simulink model "simulationSprint2"  (R2018b)
settings: Solver=FixedStepAuto  StartTime=0.0  StopTime=10  FixedStep=0.01  MaxStep=100e-3  RelTol=1e-3
(part 2 of 3)

== stateflow chart simulationSprint2/Req6 and Req 7 ==
  note: The module responsible by test the requeriment six and seven.
      |
      | Notice : i_ means input signals
      | 		o_ means output signals
      |
      | Input :
      | i_enable - Start the test. 1- Start test . 0 - Do nothing.
      | i_desiredTest - Test Number Value. All the modules recieve the
      | signal and decide either execute the test. Ex: Value "1" means that will being testing the requeriment 1.
      | i_HeadLamp - State the Head Lamp. 1 - Light On ; 0 - Light Off.
      |
      |
      | Output :
      | o_TestResult - Result of test. 1 - Test ran correctly ; 2 - Test ran incorrectly.
      | o_TestDone - Test has been completed. 1 - Completed ;
      | o_keyfob - Signal that indicates if the key is inside or not from the car. 1 - Key inside ; 0 - Key outside.
      | o_keyCommand - Signal to lock or unlock the car. "1 - lock the car ; 0 - Unlock the car" ;  -1 - Do nothing.
      | o_startButtom - Signal to start or off the car. 1- Car Start ; 0 - Car off.
      | o_gear = gear State ; 1 - Park ; 0 - Engaged.
      | o_Door = Signal to generate the open or close door. 1 - Open Door ; 0 - Close Door.
  state state_OverHeadTest1
    during:
    o_keyCommand = 0;
    o_keyfob =1 ;
    o_gear = 1 ;
    o_door = 0;
    on after(100,msec):
    o_startButtom = 1;
    on after(2.5,sec):
    r_aux=1;
    exit :
    r_aux=0;
  state state_OverHeadTest
    during:
    o_keyCommand = 0;
    o_keyfob =1 ;
    o_startButtom = 0;
    on after(600,msec):
    r_aux=1;
    exit :
    r_aux=0;
  state state_OverHeadTest2
    during:
    o_startButtom = 0;
    on after(100,msec):
    o_keyCommand = 0;
    o_keyfob =1;
    on after(200,msec):
    r_aux=1;
    exit :
    r_aux=0;
    o_keyfob =0;
  state state_OverHeadTestReq7 [commented out]
    entry :
    r_aux2 = 0;
    r_aux=0;
    during:
    on after(2,sec):
    o_gear = 1 ;
    on after(2.2,sec):
    o_keyfob =1;
    on after(2.3,sec):
    o_keyCommand = 0;
    o_startButtom = 1;
    on after(2.8,sec):
    o_startButtom = 0;
    o_keyfob =0;
    on after(5.5,sec):
    r_aux2 = 1;
    on after(10,sec):
    r_aux=1;
    exit :
    r_aux=0;
    r_aux2=0;
  state state_idle
    during:
    r_aux =0;
    o_startButtom = 0;
    o_keyCommand = 1;
    o_keyfob =0;
  state State_error
    during:
    o_TestResult =0;
    o_testDone =1 ;
    on after(100,msec):
    r_aux =1;
    exit :
    r_aux =0;
  state State_feat_ok
    during:
    o_TestResult =1;
    o_testDone =1;
    on after(10,msec):
    r_aux =1;
    exit:
    r_aux =0;
  state status_req7
    during :
    on after(1,sec):
    if(i_HeadLamp ==0 )
    r_aux = 1;
    end
    exit :
    r_aux = 0;
  state state_update
    entry:
    r_aux = 0;
    during:
    o_TestResult =0;
    o_testDone = 0;
    r_aux =1 ;
    exit:
  (default) -> state_idle
  state_OverHeadTest -> state_OverHeadTest1 [order 2] : [r_aux==1 && i_HeadLamp==1 ]
  state_OverHeadTest1 -> state_OverHeadTest2 [order 2] : [r_aux==1 && i_HeadLamp==0]
  state_idle -> state_OverHeadTest : [i_enable ==1 && (i_DesiredTest==6 || i_DesiredTest==7)]
  state_update -> state_idle : [r_aux ==1]
  state_OverHeadTest1 -> State_error [order 1] : [r_aux==1 && i_HeadLamp==1]
  state_OverHeadTest -> State_error [order 1] : [r_aux==1 && i_HeadLamp==0 ]
  state_OverHeadTest2 -> status_req7 : [r_aux==1 && i_HeadLamp==0]
  status_req7 -> State_error [order 1] : [~after(10,sec) && r_aux==1]
  State_error -> state_update : [r_aux==1]
  State_feat_ok -> state_update : [r_aux==1]
  status_req7 -> State_feat_ok [order 2] : [after(10.5,sec) && i_HeadLamp ==0  ]
  data: i_enable input; i_DesiredTest input; o_TestResult output; o_testDone output; r_aux local; i_HeadLamp input; o_keyCommand output; o_keyfob output; o_startButtom output; r_aux2 local; o_gear output; o_door output

== stateflow chart simulationSprint2/Req9 ==
  note: The module responsible by test the requeriment nine.
      |
      | Notice : i_ means input signals
      | 		o_ means output signals
      |
      | Input :
      | i_enable - Start the test. 1- Start test . 0 - Do nothing.
      | i_desiredTest - Test Number Value. All the modules recieve the
      | signal and decide either execute the test. Ex: Value "1" means that will being testing the requeriment 1.
      | i_MotorState. 1 - On ; 0 - Off .
      |
      |
      | Output :
      | o_TestResult - Result of test. 1 - Test ran correctly ; 2 - Test ran incorrectly.
      | o_TestDone - Test has been completed. 1 - Completed ;
      | o_keyfob - Signal that indicates if the key is inside or not from the car. 1 - Key inside ; 0 - Key outside.
      | o_keyCommand - Signal to lock or unlock the car. "1 - lock the car ; 0 - Unlock the car" ;  -1 - Do nothing.
      | o_startButtom - Signal to start or off the car. 1- Car Start ; 0 - Car off.
      | o_gear = gear State ; 1 - Park ; 0 - Engaged.
  state state_testTurnOnCar
    during:
    o_keyfobcommand = 0;
    o_keyfob =1;
    o_gear = 1;
    on after(1,sec):
    o_startButtom = 1;
    on after(2,sec):
    r_aux=1;
    exit:
    r_aux = 0 ;
    o_startButtom = 0;
  state state_idle
    entry :
    r_aux = 0 ;
    o_keyfobcommand = 0;
    o_keyfob =0;
    o_gear = 0;
    on after(100,msec):
    o_startButtom = 0;
  state state_testTurnOffCar
    during:
    on after (100,msec):
    o_keyfob =0;
    o_keyfobcommand = 0;
    o_keyfob =0;
    o_gear = 1;
    on after(1.1,sec):
    o_startButtom = 1;
    on after(2,sec):
    r_aux=1;
    exit:
    r_aux = 0 ;
    o_startButtom = 0;
    o_keyfob =0;
  state State_error
    entry :
    during:
    o_TestResult =0;
    o_testDone =1 ;
    on after(200,msec):
    r_aux =1;
    exit :
    r_aux =0;
  state State_feat_ok
    entry :
    during:
    o_TestResult =1;
    o_testDone =1;
    o_startButtom=0;
    on after(200,msec):
    r_aux =1;
    exit:
    r_aux =0;
  state state_update
    entry:
    r_aux = 0;
    during:
    on after(1,sec):
    o_TestResult =0;
    o_testDone = 0;
    r_aux =1 ;
    exit:
  (default) -> state_idle
  state_idle -> state_testTurnOnCar : [i_enable==1 && i_desiredTest == 9 ]
  state_update -> state_idle : [r_aux ==1]
  state_testTurnOnCar -> State_error [order 2] : [r_aux==1 && i_motorState==0]
  state_testTurnOnCar -> state_testTurnOffCar [order 1] : [r_aux==1 && i_motorState==1]
  state_testTurnOffCar -> State_error [order 2] : [r_aux==1 && i_motorState==1]
  state_testTurnOffCar -> State_feat_ok [order 1] : [r_aux==1 && i_motorState==0]
  State_error -> state_update : [r_aux==1]
  State_feat_ok -> state_update : [r_aux==1]
  data: i_enable input size=1; i_desiredTest input int8 size=1; o_TestResult output int8 size=1; o_testDone output int8 size=1; r_aux local; i_motorState input int8 size=1; o_gear output int8 size=1; o_keyfob output int8 size=1; o_keyfobcommand output int8 size=1; o_startButtom output int8 size=1

== stateflow chart simulationSprint2/Req10 ==
  note: The module responsible by test the requeriment ten.
      |
      | Notice : i_ means input signals
      | 		o_ means output signals
      |
      | Input :
      | i_enable - Start the test. 1- Start test . 0 - Do nothing.
      | i_desiredTest - Test Number Value. All the modules recieve the
      | signal and decide either execute the test. Ex: Value "1" means that will being testing the requeriment 1.
      | i_RearLamps. 1 - Light On ; 0 - Light Off .
      |
      |
      | Output :
      | o_TestResult - Result of test. 1 - Test ran correctly ; 2 - Test ran incorrectly.
      | o_TestDone - Test has been completed. 1 - Completed ;
      | o_keyfob - Signal that indicates if the key is inside or not from the car. 1 - Key inside ; 0 - Key outside.
      | o_keyCommand - Signal to lock or unlock the car. "1 - lock the car ; 0 - Unlock the car" ;  -1 - Do nothing.
      | o_brake. 1- Breaking. 0 - Not Breaking.
  state state_RearLampCarOff
    entry :
    r_aux=0;
    during :
    o_keyfobcom = 0 ;
    o_keyfob = 0 ;
    on after(200,msec):
    o_brake =1 ;
    on after(600,msec):
    r_aux=1;
    exit:
    r_aux =0 ;
  state state_RearLampCarOn
    entry :
    r_aux=0;
    o_brake=0;
    during :
    o_keyfobcom = 0 ;
    o_keyfob = 1 ;
    on after(200,msec):
    o_brake =1 ;
    on after(700,msec):
    r_aux=1;
    exit:
    r_aux =0 ;
    o_brake =0 ;
    o_keyfob = 0 ;
  state state_idle
    entry :
    r_aux=0;
  state State_error
    during:
    o_TestResult =0;
    o_testDone =1 ;
    on after(100,msec):
    r_aux =1;
    exit :
    r_aux =0;
  state State_feat_ok
    during:
    o_TestResult =1;
    o_testDone =1;
    on after(100,msec):
    r_aux =1;
    exit:
    r_aux =0;
  state state_update
    entry:
    r_aux = 0;
    on after(500,msec):
    during:
    o_TestResult =0;
    o_testDone = 0;
    r_aux =1 ;
    exit:
  (default) -> state_idle
  state_idle -> state_RearLampCarOff : [i_enable==1 && i_desiredTest==10]
  state_RearLampCarOff -> state_RearLampCarOn [order 1] : [r_aux==1 && i_RearLamps==0]
  state_RearLampCarOff -> State_error [order 2] : [r_aux==1 && i_RearLamps==1]
  state_update -> state_idle : [r_aux==1]
  state_RearLampCarOn -> State_error [order 2] : [r_aux==1 && i_RearLamps==0]
  state_RearLampCarOn -> State_feat_ok [order 1] : [r_aux==1 && i_RearLamps==1]
  State_error -> state_update : [r_aux==1]
  State_feat_ok -> state_update : [r_aux==1]
  data: i_enable input; i_desiredTest input; i_RearLamps input; o_TestResult output; o_testDone output; r_aux local; o_brake output; o_keyfob output; o_keyfobcom output

== stateflow chart simulationSprint2/Req12 ==
  note: The module responsible by test the requeriment twelve.
      |
      | Notice : i_ means input signals
      | 		o_ means output signals
      |
      | Input :
      | i_enable - Start the test. 1- Start test . 0 - Do nothing.
      | i_desiredTest - Test Number Value. All the modules recieve the
      | signal and decide either execute the test. Ex: Value "1" means that will being testing the requeriment 1.
      | i_IPCInd. 0 - Showing nothing ; 1 - Showing items .
      | i_batteryLevel . Containg the battery level value. Range = 0 - 100 %
      | i_batterySocWarning. Warning of low Battery level . If the battery value for less than or equal to 10%
      |
      | Output :
      | o_TestResult - Result of test. 1 - Test ran correctly ; 2 - Test ran incorrectly.
      | o_TestDone - Test has been completed. 1 - Completed ;
      | o_keyfob - Signal that indicates if the key is inside or not from the car. 1 - Key inside ; 0 - Key outside.
      | o_keyCommand - Signal to lock or unlock the car. "1 - lock the car ; 0 - Unlock the car" ;  -1 - Do nothing.
      | o_doorCom - Signal to represent the opening the door. 1 - Opening ; 0 - Closing ; -1 - Do nothing.
  state state_ipcoff
    during :
    o_keyfobcom = 0;
    o_keyfob = 0;
    on after(200,msec):
    r_aux=1;
    exit:
    r_aux =0;
  state state_idle
    entry:
    r_aux=0;
  state state_ipcOn
    during :
    o_keyfobcom = 0;
    o_keyfob = 1;
    on after(500,msec):
    o_doorCom = 1;
    on after(1,sec):
    r_aux=1;
    exit:
    r_aux =0;
    o_doorCom = 0;
  state State_error
    during:
    o_TestResult =0;
    o_testDone =1 ;
    on after(300,msec):
    r_aux =1;
    exit :
    r_aux =0;
    o_keyfob = 0;
  state state_batteryLevel
    during :
  state State_feat_ok
    entry :
    o_keyfob = 0;
    during:
    o_TestResult =1;
    o_testDone =1;
    on after(500,msec):
    r_aux =1;
    exit:
    r_aux =0;
    o_keyfob = 0;
  state state_update
    entry:
    r_aux = 0;
    during:
    on after(200,msec):
    o_TestResult =0;
    o_testDone = 0;
    r_aux =1 ;
    exit:
  (default) -> state_idle
  state_idle -> state_ipcoff : [i_enable==1 && i_desiredTest == 12 ]
  state_ipcoff -> State_error [order 2] : [r_aux==1 && i_IPCInd==1]
  state_update -> state_idle : [r_aux==1]
  state_ipcoff -> state_ipcOn [order 1] : [r_aux==1 && i_IPCInd==0]
  state_ipcOn -> State_error [order 2] : [r_aux==1 && i_IPCInd==0]
  State_error -> state_update : [r_aux==1]
  state_batteryLevel -> State_error [order 2] : [((i_batteryLevel <=10 && i_batterySocWarning==0 ) || (i_batteryLevel >10 && i_batterySocWarning==1 )) && after(500,msec)  ]
  state_ipcOn -> state_batteryLevel [order 1] : [r_aux==1 && i_IPCInd==1]
  state_batteryLevel -> State_feat_ok [order 1] : [((i_batteryLevel <=10 && i_batterySocWarning==1 ) || (i_batteryLevel >10 && i_batterySocWarning==0 )) && after(500,msec)  ]
  State_feat_ok -> state_update : [r_aux==1]
  data: i_enable input; i_desiredTest input; o_TestResult output; o_testDone output; r_aux local; i_IPCInd input; o_keyfob output; o_keyfobcom output; o_doorCom output; i_batteryLevel output; i_batterySocWarning input

== stateflow chart simulationSprint2/Req13 ==
  note: The module responsible by test the requeriment thirteen.
      |
      | Notice : i_ means input signals
      | 		o_ means output signals
      |
      | Input :
      | i_enable - Start the test. 1- Start test . 0 - Do nothing.
      | i_desiredTest - Test Number Value. All the modules recieve the
      | signal and decide either execute the test. Ex: Value "1" means that will being testing the requeriment 1.
      | i_ajarDoor. 1 - Door in aja state  ; 0 -  Door not in aja state .
      |
      |
      | Output :
      | o_TestResult - Result of test. 1 - Test ran correctly ; 0 - Test ran incorrectly.
      | o_TestDone - Test has been completed. 1 - Completed ;
      | o_keyCommand - Signal to lock or unlock the car. "1 - lock the car ; 0 - Unlock the car" ;  -1 - Do nothing.
      | o_doorajar. Signal to represent the opening the door. 1 - Opening ; 0 - Closing ; -1 - Do nothing.
  state state_testajarDoorTrue
    during:
    o_keyfobcommand = 0;
    o_doorAjar = 1;
    on after(200,msec):
    r_aux=1;
    exit:
    r_aux=0;
  state state_testajarDoorTrue1
    during:
    o_keyfobcommand = 0;
    o_doorAjar = 0;
    on after(500,msec):
    r_aux=1
    exit:
    r_aux=0;
  state state_idle
    entry:
    r_aux=0;
    o_doorAjar = 0;
    o_keyfobcommand = 0;
  state state_testCarlock
    during:
    o_keyfobcommand = 1;
    o_doorAjar = 1;
    on after(1,sec):
    r_aux=1
    exit:
    r_aux=0;
  state State_error
    during:
    o_TestResult =0;
    o_testDone =1 ;
    on after(100,msec):
    r_aux =1;
    exit :
    r_aux =0;
    o_doorAjar = 0;
  state State_feat_ok
    during:
    o_TestResult =1;
    o_testDone =1;
    on after(100,msec):
    r_aux =1;
    exit:
    r_aux =0;
  state state_update
    entry:
    r_aux = 0;
    on after(5,msec):
    during:
    o_TestResult =0;
    o_testDone = 0;
    r_aux =1 ;
    exit:
  state_testajarDoorTrue -> state_testajarDoorTrue1 [order 2] : [r_aux==1 && i_doorAjar == 1]
  state_testajarDoorTrue -> State_error [order 1] : [r_aux==1 && i_doorAjar == 0]
  (default) -> state_idle
  state_idle -> state_testajarDoorTrue : [i_enable==1 && i_desiredTest == 13 ]
  state_testajarDoorTrue1 -> State_error [order 2] : [r_aux==1 && i_doorAjar == 1]
  state_update -> state_idle : [r_aux==1]
  state_testajarDoorTrue1 -> state_testCarlock [order 1] : [r_aux==1 && i_doorAjar == 0]
  state_testCarlock -> State_error [order 2] : [r_aux==1 && i_doorAjar == 1]
  State_error -> state_update : [r_aux==1]
  state_testCarlock -> State_feat_ok [order 1] : [r_aux==1 && i_doorAjar == 0]
  State_feat_ok -> state_update : [r_aux==1]
  data: i_enable input; i_desiredTest input; i_doorAjar input; o_TestResult output; o_testDone output; r_aux local; o_doorAjar output int8; o_keyfobcommand output

== stateflow chart simulationSprint2/Req15 ==
  note: The module responsible by test the requeriment fifteen.
      |
      | Notice : i_ means input signals
      | 		o_ means output signals
      |
      | Input :
      | i_enable - Start the test. 1- Start test . 0 - Do nothing.
      | i_desiredTest - Test Number Value. All the modules recieve the
      | signal and decide either execute the test. Ex: Value "1" means that will being testing the requeriment 1.
      | i_gear -  geared State ; 1 - Park ; 0 - Engaged.
      | i_MotorStatus. 1 - On ; 0 - Off .
      |
      |
      | Output :
      |
      | o_TestResult - Result of test. 1 - Test ran correctly ; 0 - Test ran incorrectly.
      | o_TestDone - Test has been completed. 1 - Completed ;
      | o_keyComm - Signal to lock or unlock the car. "1 - lock the car ; 0 - Unlock the car" ;  -1 - Do nothing.
      | o_startButtom - Signal to start or off the car. 1- Car Start ; 0 - Car off.
      | o_keyfob - Signal that indicates if the key is inside or not from the car. 1 - Key inside ; 0 - Key outside.
      | o_gear = gear State ; 1 - Park ; 0 - Engaged.
  state state_gearParkOffCar
    entry:r_aux=0;
    during:
    o_keyfobcom = 0;
    on after(200,msec):
    o_keyfob =1;
    o_gear=1;
    on after(1,sec):
    o_startButtom =1;
    on after(2,sec):
    r_aux=1;
    exit :
    r_aux=0;
  state state_idle
    entry:
    r_aux=0;
  state State_error
    during:
    o_TestResult =0;
    o_testDone =1 ;
    on after(200,msec):
    r_aux =1;
    exit :
    r_aux =0;
  state state_gearParkOnCar
    entry:r_aux=0;
    during:
    o_keyfobcom = 0;
    on  after(200,msec):
    o_keyfob =1;
    o_gear=0;
    on after(400,msec):
    o_startButtom =0;
    on after(1,sec):
    r_aux=1;
    exit :
    r_aux=0;
  state state_update
    entry:
    r_aux = 0;
    on after(400,msec):
    during:
    o_TestResult =0;
    o_testDone = 0;
    r_aux =1 ;
    exit:
    o_keyfobcom = 0;
    o_keyfob =0;
    o_gear=0;
  state State_feat_ok
    during:
    o_TestResult =1;
    o_testDone =1;
    on after(200,msec):
    r_aux =1;
    exit:
    r_aux =0;
  state state_gear
    during :
    o_gear = 1;
    o_startButtom =0;
  (default) -> state_idle
  state_idle -> state_gearParkOffCar : [i_enable==1 && i_desiredTest == 15]
  state_gearParkOffCar -> state_gearParkOnCar [order 1] : [r_aux==1 && i_motorStatus==1 && i_gear ==1]
  state_gearParkOffCar -> State_error [order 2] : [(r_aux==1 && i_motorStatus==0) || (r_aux==1 && i_gear ~=1) ]
  state_update -> state_idle : [r_aux==1]
  state_gear -> State_error [order 2] : [after(500,msec) &&  i_motorStatus==1]
  state_gearParkOnCar -> State_error [order 2] : [r_aux==1 && i_motorStatus==0]
  State_error -> state_update : [r_aux==1]
  state_gearParkOnCar -> state_gear [order 1] : [r_aux==1 && i_motorStatus==1]
  state_gear -> State_feat_ok [order 1] : [after(500,msec)  && i_motorStatus==0]
  State_feat_ok -> state_update : [r_aux==1]
  data: i_enable input; i_desiredTest input; o_TestResult output; o_testDone output; r_aux local; i_motorStatus input; o_gear output; o_keyfob output; o_keyfobcom output; o_startButtom output; i_gear input

== stateflow chart simulationSprint2/Req16 ==
  note: The module responsible by test the requeriment sixteen.
      |
      | Notice : i_ means input signals
      | 		o_ means output signals
      |
      | Input :
      | i_enable - Start the test. 1- Start test . 0 - Do nothing.
      | i_desiredTest - Test Number Value. All the modules recieve the
      | signal and decide either execute the test. Ex: Value "1" means that will being testing the requeriment 1.
      | i_MotorStatus. 1 - On ; 0 - Off .
      | i_headLampLowBeam. 1 - Lamp  On ; 0 - Lamp Off.
      | i_headLampPark. 1 - Lamp On ; 0 - Lamp Off.
      | i_headLampHigh. 1 - Lamp On ; 0 - Lamp Off.
      |
      |
      | Output :
      | o_TestResult - Result of test. 1 - Test ran correctly ; 2 - Test ran incorrectly.
      | o_TestDone - Test has been completed. 1 - Completed ;
      | o_keyfobComm - Signal to lock or unlock the car. "1 - lock the car ; 0 - Unlock the car" ;  -1 - Do nothing.
      | o_headLamp - Light mode.
      | o_startButtom - Signal to start or off the car. 1- Car Start ; 0 - Car Off.
      | o_keyfob - Signal that indicates if the key is inside or not from the car. 1 - Key inside ; 0 - Key outside.
      | o_levelluminosity - Luminosity Level. Range 0 ~ 4.
  state StateTurnOnCar
    during :
    o_keyfobCom = 0;
    on after(50,msec):
    o_keyfob = 1;
    on after(100,msec):
    o_gear = 1;
    o_headLamp = 0;
    on after(150,msec):
    o_startButtom = 1;
  state state_tryTurnDown_Car
    during :
    o_startButtom = 0;
  state state_tryTurnDown_Car2
    during :
    o_headLamp = 0;
  state stateTurnOnHeadLamp
    during :
    o_headLamp = 1;
  state state_idle1
    entry:
    r_aux=0;
    o_keyfob = 0 ;
    o_levelluminosity = 4;
  state State_error1
    during:
    o_TestResult =0;
    o_testDone =1 ;
    on after(200,msec):
    r_aux =1;
    exit :
    r_aux =0;
  state state_update1
    entry:
    r_aux = 0;
    on after(200,msec):
    during:
    o_TestResult =0;
    o_testDone = 0;
    r_aux =1 ;
    exit:
    o_keyfob = 0;
    o_keyfobCom = 0;
    o_headLamp=0;
    o_startButtom = 0;
  state State_feat_ok1
    during:
    o_TestResult =1;
    o_testDone =1;
    on after(200,msec):
    r_aux =1;
    exit:
    r_aux =0;
  (default) -> state_idle1
  state_tryTurnDown_Car -> state_tryTurnDown_Car2 [order 2] : [after(1,sec) && i_motorStatus ==1]
  StateTurnOnCar -> stateTurnOnHeadLamp [order 2] : [after(300,msec) && i_motorStatus==1]
  stateTurnOnHeadLamp -> state_tryTurnDown_Car [order 1] : [after(100,msec) && i_headLampPark == 1 && i_headLampLowBeam == 0 ]
  state_update1 -> state_idle1 : [r_aux==1]
  state_idle1 -> StateTurnOnCar : [i_enable==1 && i_desiredTest ==16]
  stateTurnOnHeadLamp -> State_error1 [order 2] : [after(100,msec) && i_headLampPark ~= 1 && i_headLampLowBeam ~= 0 ]
  state_tryTurnDown_Car2 -> State_error1 [order 2] : [after(500,msec) && i_motorStatus ==1]
  state_tryTurnDown_Car2 -> State_feat_ok1 [order 1] : [after(500,msec) && i_motorStatus ==0]
  state_tryTurnDown_Car -> State_error1 [order 1] : [after(1,sec) && i_motorStatus ==0]
  StateTurnOnCar -> State_error1 [order 1] : [after(300,msec) && i_motorStatus==0]
  State_error1 -> state_update1 : [r_aux==1]
  State_feat_ok1 -> state_update1 : [r_aux==1]
  data: i_enable input; i_desiredTest input; o_TestResult output; o_testDone output; r_aux local; o_keyfobCom output; o_startButtom output; o_keyfob output; o_headLamp output; i_motorStatus input; i_headLampPark input; i_headLampLowBeam input; i_headLampHigh input; o_levelluminosity output double; o_gear output

== stateflow chart simulationSprint2/Req17 ==
  note: The module responsible by test the requeriment seventeen.
      |
      | Notice : i_ means input signals
      | 		o_ means output signals
      |
      | Input :
      | i_enable - Start the test. 1- Start test . 0 - Do nothing.
      | i_desiredTest - Test Number Value. All the modules recieve the
      | signal and decide either execute the test. Ex: Value "1" means that will being testing the requeriment 1.
      | i_lampValue. 1- Turn Lamp On ; 0 - Turn Lamp Off .
      |
      |
      | Output :
      | o_TestResult - Result of test. 1 - Test ran correctly ; 2 - Test ran incorrectly.
      | o_TestDone - Test has been completed. 1 - Completed ;
      | o_keyfobComm - Signal to lock or unlock the car. "1 - lock the car ; 0 - Unlock the car" ;  -1 - Do nothing.
      | o_keyfob - Signal that indicates if the key is inside or not from the car. 1 - Key inside ; 0 - Key outside.
  state state_testBlinkUnlockTheCar
    entry: r_aux = 0;
    during :
    on after(5,sec):
    o_keyfobcom = 0;
    on after(5.1,sec):
    if (i_lamp_value ~=r_lamp_value )
    r_blink = r_blink +1;
    r_lamp_value = i_lamp_value ;
    end
    exit:
    r_blink  = 0;
  state state_idle
    entry:
    r_aux=0;
    r_lamp_value = i_lamp_value ;
    o_ketfob = 0;
    o_keyfobcom = 1;
    r_blink = 0;
  state state_testBlinkUnlockTheCar1
    entry: r_aux = 0;
    r_lamp_value = i_lamp_value;
    during :
    o_keyfobcom = 1;
    if (i_lamp_value ~=r_lamp_value )
    r_blink = r_blink +1;
    r_lamp_value = i_lamp_value ;
    end
  state State_feat_ok
    during:
    o_TestResult =1;
    o_testDone =1;
    on after(200,msec):
    r_aux =1;
    exit:
    r_aux =0;
  state State_error
    during:
    o_TestResult =0;
    o_testDone =1 ;
    on after(200,msec):
    r_aux =1;
    exit :
    r_aux =0;
  state state_update
    entry:
    r_aux = 0;
    on after(500,msec):
    during:
    o_TestResult =0;
    o_testDone = 0;
    r_aux =1 ;
    exit:
    o_keyfobcom = 0;
  (default) -> state_idle
  state_idle -> state_testBlinkUnlockTheCar : [i_enable==1 && i_desiredTest ==17  ]
  state_testBlinkUnlockTheCar -> state_testBlinkUnlockTheCar1 [order 1] : [after(30,sec) && r_blink==2]
  state_update -> state_idle : [r_aux==1]
  state_testBlinkUnlockTheCar -> State_error [order 2] : [after(26,sec) && r_blink~=2]
  state_testBlinkUnlockTheCar1 -> State_error [order 2] : [after(40,sec) && r_blink~=4]
  state_testBlinkUnlockTheCar1 -> State_feat_ok [order 1] : [after(40,sec) && r_blink==4]
  State_feat_ok -> state_update : [r_aux==1]
  State_error -> state_update : [r_aux==1]
  data: i_enable input int8; i_desiredTest input int8; o_TestResult output int8; o_testDone output int8; r_aux local; r_blink local; r_lamp_value local; i_lamp_value input int8; o_ketfob output int8; o_keyfobcom output int8

== stateflow chart simulationSprint2/Req18 ==
  note: The module responsible by test the requeriment nineteen.
      |
      | Notice : i_ means input signals
      | 		o_ means output signals
      |
      | Input :
      | i_enable - Start the test. 1- Start test . 0 - Do nothing.
      | i_desiredTest - Test Number Value. All the modules recieve the
      | signal and decide either execute the test. Ex: Value "1" means that will being testing the requeriment 1.
      | Car Lock State. 1- Unlock ; 0 - Lock .
      |
      |
      | Output :
      | o_TestResult - Result of test. 1 - Test ran correctly ; 2 - Test ran incorrectly.
      | o_TestDone - Test has been completed. 1 - Completed ;
      | o_keyfobComm - Signal to lock or unlock the car. "1 - lock the car ; 0 - Unlock the car" ;  -1 - Do nothing.
  state state_DrlOn
    entry :
    r_aux=0;
    during :
    on after(20,sec):
    o_keyfobcom = 0;
    on after(40,sec):
    r_aux = 1 ;
    exit :
    r_aux = 0;
  state state_DrlOff
    entry : r_aux=0;
    during :
    o_keyfobcom =1;
    on after(40,sec):
    r_aux = 1 ;
    exit :
    r_aux = 0 ;
  state state_idle
    entry:
    r_aux=0;
    o_keyfobcom = 1;
  state State_feat_ok
    during:
    o_TestResult =1;
    o_testDone =1;
    on after(200,msec):
    r_aux =1;
    exit:
    r_aux =0;
  state State_error
    during:
    o_TestResult =0;
    o_testDone =1 ;
    on after(200,msec):
    r_aux =1;
    exit :
    r_aux =0;
  state state_update
    entry:
    r_aux = 0;
    on after(300,msec):
    during:
    o_TestResult =-1;
    o_testDone = 0;
    r_aux =1 ;
    exit:
  (default) -> state_idle
  state_idle -> state_DrlOn : [i_enable==1 && i_desiredTest == 18 ]
  state_DrlOn -> state_DrlOff [order 1] : [r_aux==1 && i_DRL==1]
  state_DrlOn -> State_error [order 2] : [r_aux==1 && i_DRL==0]
  state_DrlOff -> State_error [order 2] : [r_aux==1 && i_DRL==1]
  state_DrlOff -> State_feat_ok [order 1] : [r_aux==1 && i_DRL==0]
  state_update -> state_idle : [r_aux==1]
  State_feat_ok -> state_update : [r_aux==1]
  State_error -> state_update : [r_aux==1]
  data: i_enable input int8; i_desiredTest input; o_TestResult output; o_testDone output; i_DRL input; r_aux local double; o_keyfobcom output

== stateflow chart simulationSprint2/"Req 2" ==
  note: The module responsible by test the requeriment one.
      |
      | Notice : i_ means input signals
      | 		o_ means output signals
      |
      | Input :
      | i_enable - Start the test. 1- Start test . 0 - Do nothing.
      | i_desiredTest - Test Number Value. All the modules recieve the
      | signal and decide either execute the test. Ex: Value "1" means that will being testing the requeriment 1.
      | i_WindowRightState = Windows State. 1- Windows Opening  ; 0 - Windows Closing ;  -1 - Do nothing.
      | i_WindowLeftState = Windows State. 1- Windows Opening  ; 0 - Windows Closing ;  -1 - Do nothing.
      | Output :
      | o_keyfob - Signal that indicates if the key is inside or not from the car. 1 - Key inside ; 0 - Key outside.
      | o_startButtom - Signal to start or off the car. 1- Car Start ; 0 - Car off.
      | o_WindowValue - Signal to move the windows " 1 - Opening ; 0- Closing ; -1 - Do Nothing  ;
      | o_gear = gear State ; 1 - Park ; 0 - Engaged.
      | o_keyfobCommand - Signal to lock or unlock the car. "1 - lock the car ; 0 - Unlock the car" ;  -1 - Do nothing.
      | o_TestResult - Result of test. 1 - Test ran correctly ; 2 - Test ran incorrectly.
      | o_TestDone - Test has been completed. 1 - Completed ;
  state State_idle
    exit :
    r_aux=0;
    r_count = 1 ;
    r_error = 0;
    o_startButtom = 0;
    o_keyfobCommand = 2;
    o_gear = 0 ;
    o_keyfob=0;
    o_WindowValue = -1;
  state state_readyingSystem
    during:
    on after (50,msec):
    o_keyfob =1;
    o_keyfobCommand = 0 ;
    o_gear = 1 ;
    on after(0.5,sec):
    o_startButtom = 1;
    on after(1.5,sec):
    r_aux=1;
    exit :
    r_aux=0;
  state state_testCarOn
    during:
    o_WindowValue =0 ;
    on after(2,sec):
    r_aux=1;
    exit :
    r_aux=0;
  state state_testCarOff
    during:
    o_startButtom = 0;
    on after(2,sec):
    o_WindowValue= 0;
    on after(3,sec):
    r_aux=1;
    exit :
    r_aux=0;
    o_WindowValue= -1;
  state State_error
    during:
    o_TestResult =0;
    o_testDone =1 ;
    on after(200,msec):
    r_aux =1;
    exit :
    r_aux =0;
  state state_temp
  state state_testAfter10sec
    entry:
    o_WindowValue= 0;
  state state_update
    entry:
    r_aux = 0;
    during:
    o_TestResult =0;
    o_testDone = 0;
    on after(500,msec):
    r_aux =1 ;
    exit:
  state State_feat_ok
    during:
    o_TestResult =1;
    o_testDone =1;
    on after(200,msec):
    r_aux =1;
    exit:
    r_aux =0;
  (default) -> State_idle
  State_idle -> state_readyingSystem : [i_enable==1 && i_desiredTest ==2 ]
  state_readyingSystem -> state_testCarOn : [r_aux==1]
  state_testCarOn -> state_testCarOff [order 2] : [(i_WindowRightState==0 && i_WindowLeftState == 0)  && r_aux==1]
  state_update -> State_idle : [r_aux==1]
  state_testCarOn -> State_error [order 1] : [(i_WindowRightState~=0 || i_WindowLeftState ~= 0)   && r_aux==1]
  state_testCarOff -> State_error [order 2] : [(i_WindowRightState~=0 || i_WindowLeftState ~= 0)   && r_aux==1]
  state_testAfter10sec -> State_error [order 1] : [(i_WindowRightState~=-1 && i_WindowLeftState ~= -1) && after(300,msec)]
  State_error -> state_update : [r_aux==1]
  state_testCarOff -> state_temp [order 1] : [(i_WindowRightState==0 && i_WindowLeftState == 0)  && r_aux==1]
  state_temp -> state_testAfter10sec : [after(11,sec)]
  state_testAfter10sec -> State_feat_ok [order 2] : [(i_WindowRightState==-1 && i_WindowLeftState == -1) && after(300,msec)]
  State_feat_ok -> state_update : [r_aux==1]
  data: o_TestResult output; r_aux local; i_desiredTest input; i_enable input; r_error local; o_testDone output; r_count local; o_keyfob output; i_WindowRightState input; o_keyfobCommand output; o_startButtom output; o_WindowValue output; o_gear output; i_WindowLeftState input

== stateflow chart simulationSprint2/Req 4 ==
  state state_test_unlock_doors [commented out]
    during:
    o_keyfob =1;
    o_keyfobCom = 0;
    on after(10,msec):
    o_lockDoor = 0 ;
    on after(1.5,sec):
    r_aux = 1;
    exit : r_aux = 0;
  note: The module responsible by test the requeriment four.
      |
      | Notice : i_ means input signals
      | 		o_ means output signals
      |
      | Input :
      | i_enable - Start the test. 1- Start test . 0 - Do nothing.
      | i_desiredTest - Test Number Value. All the modules recieve the
      | signal and decide either execute the test. Ex: Value "1" means that will being testing the requeriment 1.
      | i_WindowsStateAnd - And condition with the WindowState . 1-  Both is Windows Closing ; 0 - Windows Opening ;  -1 - Do nothing.
      | i_WindowsStateAnd - And condition with the DoorState. 1 - Both Door are closing  ;  0 - Some Door is opening ;  -1 Do nothing.
      | i_WindowsStateOr - Or condition with the DoorState. 1 - Some Door is closing ;  0 - Both Door are opening ;  -1 Do nothing.
      | i_stateDoorAnd - And condition with the Door Lock State. 1 - Both Door are Locked; 0 - Some Door is unlocked; -1 Do nothing.
      | i_stateDoorOR - Or condition with the Door Lock State. 1 - Some Door is locked;  0 - Both Door are unlocked ;  -1 Do nothing.
      |
      | Output :
      | o_TestResult - Result of test. 1 - Test ran correctly ; 2 - Test ran incorrectly.
      | o_TestDone - Test has been completed. 1 - Completed .
      | o_keyfob - Signal that indicates if the key is inside or not from the car. 1 - Key inside ; 0 - Key outside.
      | o_keyfobComm - Signal to lock or unlock the car. "1 - lock the car ; 0 - Unlock the car" ;  -1 - Do nothing.
      | o_WindowState - Signal to move the windows " 0 - Opening ; 1- Closing ; -1 - Do Nothing  ;
      | o_lockDoor = Lock Door ; 1 - Lock the doors; 0 - unlock the doors.
  state State_idle
    entry :
    r_aux=0;
    o_TestResult = 0;
    o_lockDoor=-1;
    during:
  state state_test_lock_doors
    during:
    o_keyfob =1;
    o_keyfobCom = 0;
    on after(200,msec):
    o_lockDoor = 1 ;
    on after(300,msec):
    o_gear =1;
    on after(400,msec):
    o_startButtom =1 ;
    on after(1.7,sec):
    r_aux = 1;
    exit : r_aux = 0;
  state state_test_windowsTest
    during:
    o_keyfob =1;
    o_keyfobCom = 0;
    on after(100,msec):
    o_startButtom =1 ;
    on after(600,msec):
    o_DDSCommand = 0;
    on after(1,sec):
    o_windowState = 0 ;
    on after(2.5,sec):
    r_aux = 1;
    exit : r_aux = 0;
  state State_error
    during:
    o_TestResult =0;
    o_testDone =1 ;
    on after(100,msec):
    r_aux =1;
    exit :
    r_aux =0;
  state state_WindowsTest1
    during:
    o_keyfob =1;
    o_keyfobCom = 0;
    on after(100,msec):
    o_startButtom =1 ;
    on after(800,msec):
    o_DDSCommand = 1;
    on after(2.4,sec):
    o_windowState = 1 ;
    on after(4,sec):
    r_aux = 1;
    exit : r_aux = 0;
  state State_feat_ok
    entry :
    o_lockDoor=0;
    o_keyfob = 0 ;
    o_keyfobCom =0;
    during:
    o_TestResult =1;
    o_testDone =1;
    on after(500,msec):
    r_aux =1;
    exit:
    r_aux =0;
  state state_update
    entry:
    o_lockDoor=0;
    o_keyfob = 0 ;
    o_keyfobCom =0;
    r_aux = 0;
    on after(500,msec):
    during:
    o_TestResult =0;
    o_testDone = 0;
  (default) -> ? [commented out] : [r_aux ==1 &&  i_stateDoorRight==0 && i_stateDoorLeft ==0]
  state_test_unlock_doors -> ? [commented out] : [r_aux ==1 &&  i_stateDoorRight ~=0 && i_stateDoorLeft ~=0]
  (default) -> State_idle
  State_idle -> state_test_lock_doors : [i_enable==1 && i_desiredTest ==4 ]
  state_test_lock_doors -> state_test_windowsTest [order 1] : [r_aux ==1 &&  i_stateDoorRight==1 && i_stateDoorLeft ==1]
  state_update -> State_idle : [after(100,msec)]
  state_test_windowsTest -> State_error [order 2] : [r_aux ==1 &&  i_windowStateLeft~=-1 && i_windowStateRight~=-1]
  state_test_lock_doors -> State_error [order 2] : [r_aux ==1 &&  i_stateDoorRight~=1 && i_stateDoorLeft ~=1]
  state_test_windowsTest -> state_WindowsTest1 [order 1] : [r_aux ==1 &&  i_windowStateLeft==-1 && i_windowStateRight==-1]
  state_WindowsTest1 -> State_error [order 2] : [r_aux ==1 &&  i_windowStateLeft~=1 && i_windowStateRight~=1]
  State_error -> state_update : [r_aux==1]
  state_WindowsTest1 -> State_feat_ok [order 1] : [r_aux ==1 &&  i_windowStateLeft==1 && i_windowStateRight==1]
  State_feat_ok -> state_update : [r_aux==1]
  data: o_TestResult output; r_aux local; i_desiredTest input; i_enable input; o_testDone output; i_stateDoorRight input; i_stateDoorLeft input; o_keyfob output; o_keyfobCom output; o_lockDoor output; o_windowState output; i_windowStateLeft input; o_startButtom output; o_DDSCommand output; i_windowStateRight input; o_gear output

== stateflow chart simulationSprint2/Req19 ==
  note: The module responsible by test the requeriment fourteen.
      |
      | Notice : i_ means input signals
      | 		o_ means output signals
      |
      | Input :
      | i_enable - Start the test. 1- Start test . 0 - Do nothing.
      | i_desiredTest - Test Number Value. All the modules recieve the
      | signal and decide either execute the test. Ex: Value "1" means that will being testing the requeriment 1.
      | i_MotorState. 1 - On ; 0 - Off .
      | i_speed - Car Speed. Range - 0 ~ 220 km/h
      | i_LeftBackDoorLockState. 1 - Door Unlock . 0 - Door Lock.
      | i_RightBackDoorLockState. 1 - Door Unlock . 0 - Door Lock.
      |
      | Output :
      | o_TestResult - Result of test. 1 - Test ran correctly ; 0 - Test ran incorrectly.
      | o_TestDone - Test has been completed. 1 - Completed ;
      | o_keyfobComm - Signal to lock or unlock the car. "1 - lock the car ; 2 - Unlock the car" ;  0 - Do nothing.
      | o_startButtom - Signal to start or off the car. 1- Car Start ; 0 - Car off.
      | o_keyfob - Signal that indicates if the key is inside or not from the car. 1 - Key inside ; 0 - Key outside.
      | o_gear = gear State ; 1 - Park ; 0 - Engaged.
  state state_gearParkOnCar
    entry:r_aux=0;
    during:
    o_keyfobcom = 2;
    on after(50,msec):
    o_keyfobcom = 0;
    on after(200,msec):
    o_keyfob =1;
    o_gear=1;
    on after(300,msec):
    o_startButtom =1;
    on after(5,sec):
    r_aux=1;
    exit :
    r_aux=0;
  state state_idle
    entry:
    r_aux=0;
    during :
    o_throttle = 0 ;
    o_epb = 0 ;
  state State_error
    during:
    o_TestResult =0;
    o_testDone =1 ;
    on after(300,msec):
    r_aux =1;
    exit :
    r_aux =0;
  state state_testSpeedmeter
    entry :
    o_epb = 0 ;
    o_throttle = 70 ;
  state state_update
    entry:
    r_aux = 0;
    on after(200,msec):
    during:
    o_TestResult =0;
    o_testDone = 0;
    r_aux =1 ;
    exit:
    o_keyfob = 0 ;
    o_keyfobcom = 0;
    o_gear = 0 ;
    o_startButtom = 0 ;
  state State_feat_ok
    during:
    o_TestResult =1;
    o_testDone =1;
    on after(100,msec):
    r_aux =1;
    exit:
    r_aux =0;
  (default) -> state_idle
  state_idle -> state_gearParkOnCar : [i_enable==1 && i_desiredTest == 19]
  state_gearParkOnCar -> state_testSpeedmeter [order 1] : [r_aux==1 && i_motorStatus==1]
  state_update -> state_idle : [r_aux==1]
  state_gearParkOnCar -> State_error [order 2] : [r_aux==1 && i_motorStatus==0]
  State_error -> state_update : [r_aux==1]
  state_testSpeedmeter -> State_error [order 2] : [after(10,sec) && (i_speed<8 || ( i_RightBackDoorLockState ~=0 || i_LeftBackDoorLockState ~=0))]
  state_testSpeedmeter -> State_feat_ok [order 1] : [(after(10,sec) &&  (i_speed > 10  ) && i_RightBackDoorLockState ==0 && i_LeftBackDoorLockState ==0)]
  State_feat_ok -> state_update : [r_aux==1]
  data: i_enable input; i_desiredTest input; o_TestResult output; o_testDone output; r_aux local; i_motorStatus input; o_gear output; o_keyfob output; o_keyfobcom output; o_startButtom output; o_throttle output; i_speed input; i_LeftBackDoorLockState input; i_RightBackDoorLockState input; o_epb output

== stateflow chart simulationSprint2/Req21 ==
  note: The module responsible by test the requeriment nine.
      |
      | Notice : i_ means input signals
      | 		o_ means output signals
      |
      | Input :
      | i_enable - Start the test. 1- Start test . 0 - Do nothing.
      | i_desiredTest - Test Number Value. All the modules recieve the
      | signal and decide either execute the test. Ex: Value "1" means that will being testing the requeriment 1.
      | i_MotorState. 1 - On ; 0 - Off .
      | i_CarLockState. 1 - Car unlock ; 0 - Car Lock.
      |
      |
      | Output :
      | o_TestResult - Result of test. 1 - Test ran correctly ; 2 - Test ran incorrectly.
      | o_TestDone - Test has been completed. 1 - Completed ;
      | o_keyfob - Signal that indicates if the key is inside or not from the car. 1 - Key inside ; 0 - Key outside.
      | o_keyCommand - Signal to lock or unlock the car. "1 - lock the car ; 2 - Unlock the car" ;  0 - Do nothing.
      | o_startButtom - Signal to start or off the car. 1- Car Start ; 0 - Car off.
      | o_gear - gear State ; 1 - Park ; 0 - Engaged.
      | o_peopleSensor - Signal that indicates if have someone in the car. 1 - Someone inside 0 - No one inside.
      | o_keyfobCode - Hash Code of the key.
      | o_doorAction - Action in the door . 1 - Opening door 0 - Closing Door
  state state_putKeyIntheCar
    during :
    o_keyfobCode = 60;
    on after(50,msec):
    o_keyfobcommand =2;
    on after(100,msec):
    o_keyfobcommand =0;
    o_doorAction = 1;
    o_keyfob = 1;
    on after(120,msec):
    o_gear = 1;
    exit :
    o_doorAction =0;
  state stateTryCarOn
    entry :
    during :
    on after(120,msec):
    o_startButtom =1 ;
    exit :
    o_startButtom =0 ;
  state state_idle
    entry :
    r_aux = 0 ;
    o_keyfobcommand = 0;
    o_keyfob =0;
    o_gear = 0;
    on after(100,msec):
    o_startButtom = 0;
  state state_LockCarwithKeyInside
    during :
    o_doorAction =1;
    on after (1,sec):
    o_doorAction =0;
    o_keyfobCode = 70
    on after(1.2,sec):
    o_keyfobcommand =1;
    on after(1.8,sec):
    o_keyfobcommand =0;
    exit :
    o_keyfob = 0;
  state state_TryCaronOtherKey
    entry :
    o_keyfobCode = 70;
    during :
    on after(500,msec):
    o_keyfobcommand =2;
    on after(900,msec):
    o_keyfobcommand =0;
    on after(1.5,sec):
  state stateTryTurnOnCarKey60
    entry :
    o_keyfobCode = 70;
    during :
    o_doorAction =1;
    on after (1,sec):
    o_doorAction =0;
    o_keyfob = 1;
    on after(100,msec):
    o_keyfobCode = 60;
    on after(1.6,sec):
    o_startButtom = 1;
  state State_error
    entry :
    during:
    o_TestResult =0;
    o_testDone =1 ;
    on after(200,msec):
    r_aux =1;
    exit :
    r_aux =0;
  state state_withValideteKey
    during:
    o_keyfobCode = 60;
    o_doorAction =1;
    on after(200,msec):
    o_doorAction =0;
    o_keyfob = 0;
    on after(500,msec):
    o_keyfobcommand =1;
    on after(600,msec):
    o_keyfobcommand =0;
  state state_update
    entry:
    r_aux = 0;
    during:
    on after(1,sec):
    o_TestResult =0;
    o_testDone = 0;
    r_aux =1 ;
    exit:
  state State_feat_ok
    during:
    o_TestResult =1;
    o_testDone =1;
    on after(100,msec):
    r_aux =1;
    exit:
    r_aux =0;
  (default) -> state_idle
  state_putKeyIntheCar -> stateTryCarOn [order 1] : [after(200,msec) && i_CarLockState==1 && i_pcmKeyCodeTest==1 ]
  stateTryCarOn -> state_LockCarwithKeyInside [order 1] : [i_MotorStatus==1 && after(800,msec)]
  state_idle -> state_putKeyIntheCar : [i_enable==1 && i_desiredTest == 21 ]
  state_LockCarwithKeyInside -> state_TryCaronOtherKey [order 1] : [i_CarLockState==0 &&  i_pcmKeyCodeTest==0  &&after(2.2,sec)]
  state_update -> state_idle : [r_aux ==1]
  stateTryCarOn -> State_error [order 2] : [i_MotorStatus==0 && after(800,msec)]
  state_TryCaronOtherKey -> State_error [order 2] : [i_CarLockState ~=1 && after(2,sec)]
  state_TryCaronOtherKey -> stateTryTurnOnCarKey60 [order 1] : [i_CarLockState ==1 && after(2,sec)]
  state_putKeyIntheCar -> State_error [order 2] : [after(130,msec) && (i_CarLockState~=1 || i_pcmKeyCodeTest~=1 ) ]
  state_LockCarwithKeyInside -> State_error [order 2] : [(i_pcmKeyCodeTest ~=0 || i_CarLockState ~=0) && after(2.2,sec)]
  stateTryTurnOnCarKey60 -> State_error [order 1] : [i_MotorStatus == 1 && after(2.2,sec) ]
  stateTryTurnOnCarKey60 -> state_withValideteKey [order 2] : [i_MotorStatus == 0 && after(2.2,sec) ]
  State_error -> state_update : [r_aux==1]
  state_withValideteKey -> State_error [order 2] : [after(1.5,sec) && i_CarLockState~=0]
  state_withValideteKey -> State_feat_ok [order 1] : [after(1.5,sec) && i_CarLockState==0]
  State_feat_ok -> state_update : [r_aux==1]
  data: i_enable input size=1; i_desiredTest input int8 size=1; o_TestResult output int8 size=1; o_testDone output int8 size=1; r_aux local; i_CarLockState input int8 size=1; o_gear output int8 size=1; o_keyfob output int8 size=1; o_keyfobcommand output int8 size=1; o_startButtom output int8 size=1; i_MotorStatus input; o_keyfobCode output; o_doorAction output; i_pcmKeyCodeTest input
